simulink model "c281x_adcpwmasynctest_ert"  (R2021b)
settings: Solver=FixedStepDiscrete  StartTime=0.0  StopTime=inf  RelTol=1e-3  EnableMultiTasking=on
undefined symbols (not defined in the file or in its folder): Asymmetric, Up
libraries: c281xlib x2, demo_controls x1, c2000lib x1
settings Model: Creator=The MathWorks, Inc.  LastModifiedBy=The MathWorks, Inc.
settings SolverCC: AlgebraicLoopSolver=TrustRegion
settings DataIOCC: LimitDataPoints=on  SaveFormat=Array  SaveOutput=off  SaveTime=off  ReturnWorkspaceOutputs=off
settings OptimizationCC: ExpressionDepthLimit=2147483647  InitFltsAndDblsToZero=on  LifeSpan=1  MaxStackSize=64  EfficientTunableParamExpr=on
settings DebuggingCC: UnderspecifiedInitializationDetection=Classic  MergeDetectMultiDrivingBlocksExec=none  SignalResolutionControl=TryResolveAllWithWarning  InheritedTsInSrcMsg=none  MultiTaskDSMMsg=warning  MultiTaskCondExecSysMsg=none  FcnCallInpInsideContextMsg=warning  AllowSymbolicDim=off  StateNameClashWarn=warning  SFUnexpectedBacktrackingDiag=warning  SFNoUnconditionalDefaultTransitionDiag=warning  SFExecutionAtInitializationDiag=none  SFMachineParentedDataDiag=warning  ArithmeticOperatorsInVariantConditions=warning
settings HardwareCC: ProdBitPerChar=16  ProdBitPerInt=16  ProdBitPerPointer=32  ProdBitPerSizeT=32  ProdBitPerPtrDiffT=32  ProdLargestAtomicInteger=Integer  ProdLargestAtomicFloat=None  ProdWordSize=16  ProdHWDeviceType=Texas Instruments->C2000  TargetBitPerChar=16  TargetBitPerInt=16  TargetBitPerPointer=16  TargetLargestAtomicInteger=Integer  TargetIntDivRoundTo=Zero  TargetEndianess=LittleEndian  TargetWordSize=16  TargetHWDeviceType=Texas Instruments->C2000  ProdEqTarget=off
settings ModelReferenceCC: PropagateSignalLabelsOutOfModel=off
settings SFSimCC: SimUseLocalCustomCode=off  MATLABDynamicMemAlloc=off  CustomCodeUndefinedFunction=UseInterfaceOnly
settings RTWCC: Description=Embedded Coder  SystemTargetFile=ert.tlc  HardwareBoard=TI F281x  TemplateMakefile=ert_default_tmf  PostCodeGenCommand=; codertarget.postCodeGenHookCommand(h)  RTWUseLocalCustomCode=off  Toolchain=Texas Instruments Code Composer Studio (C2000)
settings CodeAppCC: IgnoreCustomStorageClasses=off  CustomSymbolStrType=$N$R$M  StateflowObjectComments=on  InternalIdentifier=Classic
settings ERTTargetCC: MultiwordLength=2048  ParMdlRefBuildCompliant=off  CompOptLevelCompliant=off  CPPClassGenCompliant=off  ExtModeStaticAllocSize=2048  ExtModeMexFile=TIC2000ExternalModeOpen  ExtModeIntrfLevel=Level2 - Open  ConvertIfToSwitch=off  SuppressUnreachableDefaultCases=off
settings ConfigComp: CovMetricSettings=dw  CovSaveCumulativeToWorkspaceVar=on  CovSaveSingleToWorkspaceVar=on  CovExternalEMLEnable=off  CovSFcnEnable=off

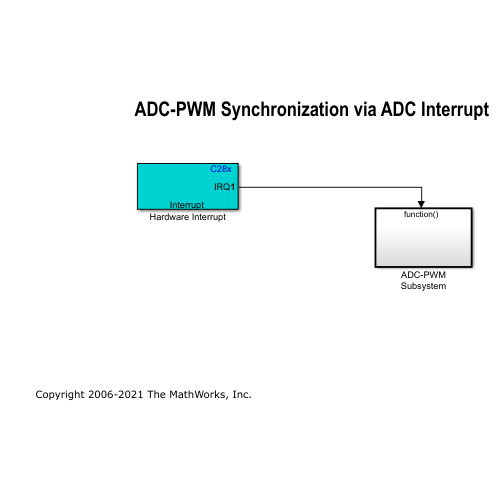
[thumbnail: Simulink's stored preview of the top-level diagram]
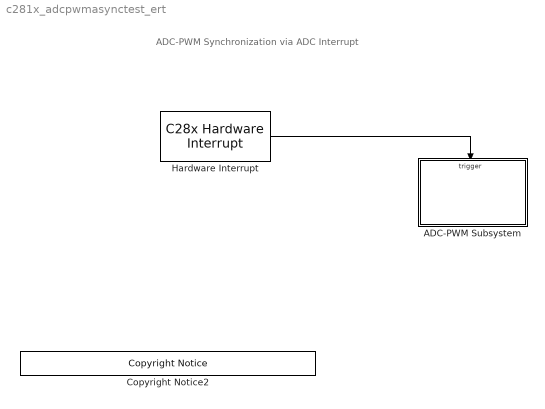
== system c281x_adcpwmasynctest_ert ==
  note: ADC-PWM Synchronization via ADC Interrupt
  ADC-PWM Subsystem : Subsystem  TreatAsAtomicUnit=on
  Copyright Notice2 : demo_controls/Copyright Notice  year=2006  prod=tic2000
      settings: SourceProductBaseCode=ME
  Hardware Interrupt : c2000lib/Scheduling/C28x Hardware Interrupt  irqnumbers=[1]  pienumbers=[6]  irqpriorities=[30]  irqpreempts=[1]  showinput=off  dspchiptype=C281X
      settings: SourceProductBaseCode=TIC2000
  wires:
  Hardware Interrupt/1 -> ADC-PWM Subsystem/Trigger

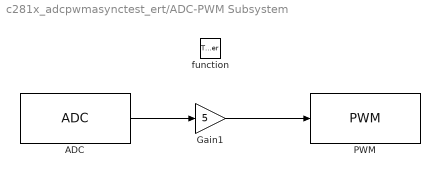
== system c281x_adcpwmasynctest_ert/ADC-PWM Subsystem ==
  function : TriggerPort  TriggerType=function-call  VariantControl=Variant
  ADC : c281xlib/ADC  useModule=A  useMode=Sequential  sourceSOC=EVA  sourceSOCA=EVA  sourceSOCB=Software  Ts=-1  dType=uint16  postInterrupt=on  numConversionsSingle=1  numConversionsDouble=1  conv0=ADCINB0  conv1=ADCINB1  conv2=ADCINB2  conv3=ADCINB3  conv4=ADCINA4  conv5=ADCINA5  conv6=ADCINB6  conv7=ADCINA7  conv8=ADCINB0  conv9=ADCINB1  conv10=ADCINB2  conv11=ADCINB3  conv12=ADCINB4  conv13=ADCINB5  conv14=ADCINB6  conv15=ADCINB7  convAB0=ADCINA0 and ADCINB0  convAB1=ADCINA1 and ADCINB1  convAB2=ADCINA5 and ADCINB5  convAB3=ADCINA1 and ADCINB1  convAB4=ADCINA1 and ADCINB1  convAB5=ADCINA1 and ADCINB1  convAB6=ADCINA1 and ADCINB1  convAB7=ADCINA1 and ADCINB1  convA0=ADCINA0  convA1=ADCINA1  convA2=ADCINA2  convA3=ADCINA3  convA4=ADCINA4  convA5=ADCINA5  convA6=ADCINA6  convA7=ADCINA7  convB0=ADCINB0  convB1=ADCINB1  convB2=ADCINB2  convB3=ADCINB3  convB4=ADCINB4  convB5=ADCINB5  convB6=ADCINB6  convB7=ADCINB7  c28xmultiPort=off
      settings: SourceProductBaseCode=TIC2000
  Gain1 : Gain  Gain=5  OutDataTypeStr=Inherit: Same as input  ParamDataTypeStr=Inherit: Same as input
  PWM : c281xlib/PWM  useModule=A  timerSource=Specify via dialog  timerPeriod=20480  waveformType=Asymmetric(Up)  periodUnits=Clock cycles  preScaler=1/128  unit1Status=on  unit1Source=Input port  unit1Value=18500  unit2Status=off  unit2Source=Specify via dialog  unit2Value=18500  unit3Status=off  unit3Source=Specify via dialog  unit3Value=18500  dutyCycleUnits=Clock cycles  logicSource=Specify via dialog  unit1_1Logic=Active high  unit1_2Logic=Active low  unit2_1Logic=Active high  unit2_2Logic=Active low  unit3_1Logic=Active high  unit3_2Logic=Active low  enableDeadband1=off  enableDeadband2=off  enableDeadband3=off  deadbandPrescaler=1  deadbandPeriodSource=Specify via dialog  deadbandPeriod=1  adcStartTrigger=Period match  adcstartEvent=None
      settings: SourceProductBaseCode=TIC2000
  wires:
  ADC/1 -> Gain1/1
  Gain1/1 -> PWM/1
